simulink model "implementation_deploy_simulador"  (R2024b)
settings: configuration reference "Configuration" (kept outside this file)
undefined symbols (not defined in the file): aceleracao_lateral_max, constans_PID, desired_x, desired_y, DiscIntNeverNeededParam, max_velocity_longitudinal, pos_theta, pos_x, pos_y, vel_x
libraries: ros2lib x4, simulink_extras x1, drivingvehiclecontroller x1, slpidlib x1
settings Model: DataDictionary=mplementacao_deploy_simulador.sldd  Creator=helenamandl  LastModifiedBy=thailon
settings ConfigSetRef: SourceName=Configuration

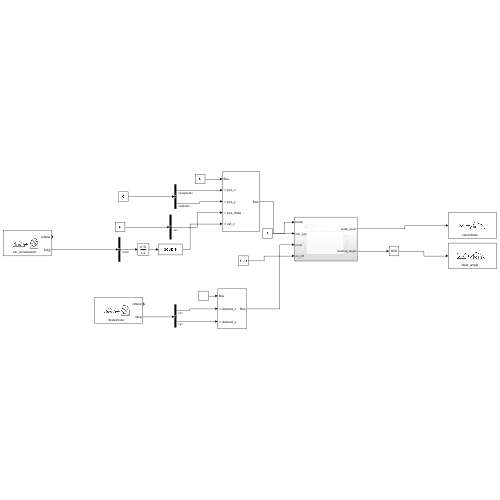
[thumbnail: Simulink's stored preview of the top-level diagram]
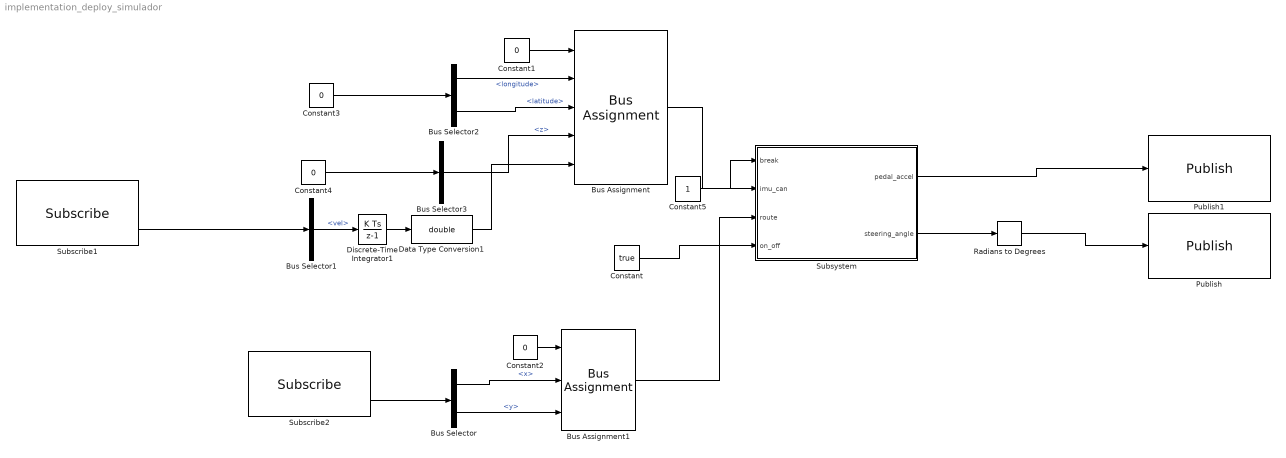
== system implementation_deploy_simulador ==
  Bus Assignment : BusAssignment  AssignedSignals=pos_x,pos_y,pos_theta,vel_x
  Bus Assignment1 : BusAssignment  AssignedSignals=desired_x,desired_y
  Bus Selector : BusSelector  OutputSignals=pose.position.x,pose.position.y
  Bus Selector1 : BusSelector  OutputSignals=vel
  Bus Selector2 : BusSelector  OutputSignals=longitude,latitude
  Bus Selector3 : BusSelector  OutputSignals=z
  Constant : Constant  Value=true  OutDataTypeStr=boolean
  Constant1 : Constant  Value=0  OutDataTypeStr=Bus: bus_imu
  Constant2 : Constant  Value=0  OutDataTypeStr=Bus: bus_route
  Constant3 : Constant  Value=0  OutDataTypeStr=Bus: bus_imu
  Constant4 : Constant  Value=0  OutDataTypeStr=Bus: bus_imu
  Constant5 : Constant
  Data Type Conversion1 : DataTypeConversion  OutDataTypeStr=double  SaturateOnIntegerOverflow=off  RndMeth=Floor
  Discrete-Time Integrator1 : DiscreteIntegrator  SampleTime=-1  ICPrevOutput=DiscIntNeverNeededParam  ICPrevScaledInput=DiscIntNeverNeededParam
  Publish : ros2lib/Publish  topicSource=Specify your own  topic=steer_angle  messageType=std_msgs/Float32  QOSHistory=Keep last  QOSDepth=1  QOSReliability=Reliable  QOSDurability=Volatile  QOSDeadline=Inf  QOSLifespan=Inf  QOSLiveliness=Automatic  QOSLeaseDuration=Inf  QOSAvoidROSNamespaceConventions=off
  Publish1 : ros2lib/Publish  topicSource=Specify your own  topic=velocidade  messageType=std_msgs/Float32  QOSHistory=Keep last  QOSDepth=1  QOSReliability=Reliable  QOSDurability=Volatile  QOSDeadline=Inf  QOSLifespan=Inf  QOSLiveliness=Automatic  QOSLeaseDuration=Inf  QOSAvoidROSNamespaceConventions=off
  Radians to Degrees : simulink_extras/Transformations/Radians to Degrees
  Subscribe1 : ros2lib/Subscribe  topicSource=Specify your own  topic=car_acceleration  messageType=std_msgs/Float32  sampleTime=ts_ros2  QOSHistory=Keep last  QOSDepth=10  QOSReliability=Reliable  QOSDurability=Volatile  QOSDeadline=Inf  QOSLifespan=Inf  QOSLiveliness=Automatic  QOSLeaseDuration=Inf  QOSAvoidROSNamespaceConventions=off
  Subscribe2 : ros2lib/Subscribe  topicSource=Specify your own  topic=/teste/route  messageType=geometry_msgs/PoseStamped  sampleTime=ts_ros2  QOSHistory=Keep last  QOSDepth=10  QOSReliability=Reliable  QOSDurability=Volatile  QOSDeadline=Inf  QOSLifespan=Inf  QOSLiveliness=Automatic  QOSLeaseDuration=Inf  QOSAvoidROSNamespaceConventions=off
  Subsystem : Subsystem
  wires:
  Subsystem/1(pedal_accel) -> Publish1/1
  Bus Assignment1/1 -> Subsystem/3(route)
  Constant/1 -> Subsystem/4(on_off)
  Bus Assignment/1 -> Subsystem/2(imu_can)
  Bus Selector/2 -> Bus Assignment1/3  "<y>"
  Bus Selector1/1 -> Discrete-Time Integrator1/1  "<vel>"
  Constant2/1 -> Bus Assignment1/1
  Constant5/1 -> Subsystem/1(break)
  Constant3/1 -> Bus Selector2/1
  Subscribe2/2 -> Bus Selector/1
  Subsystem/2(steering_angle) -> Radians to Degrees/1
  Constant4/1 -> Bus Selector3/1
  Data Type Conversion1/1 -> Bus Assignment/5
  Bus Selector/1 -> Bus Assignment1/2  "<x>"
  Constant1/1 -> Bus Assignment/1
  Bus Selector2/1 -> Bus Assignment/2  "<longitude>"
  Bus Selector2/2 -> Bus Assignment/3  "<latitude>"
  Bus Selector3/1 -> Bus Assignment/4  "<z>"
  Radians to Degrees/1 -> Publish/1
  Subscribe1/2 -> Bus Selector1/1
  Discrete-Time Integrator1/1 -> Data Type Conversion1/1

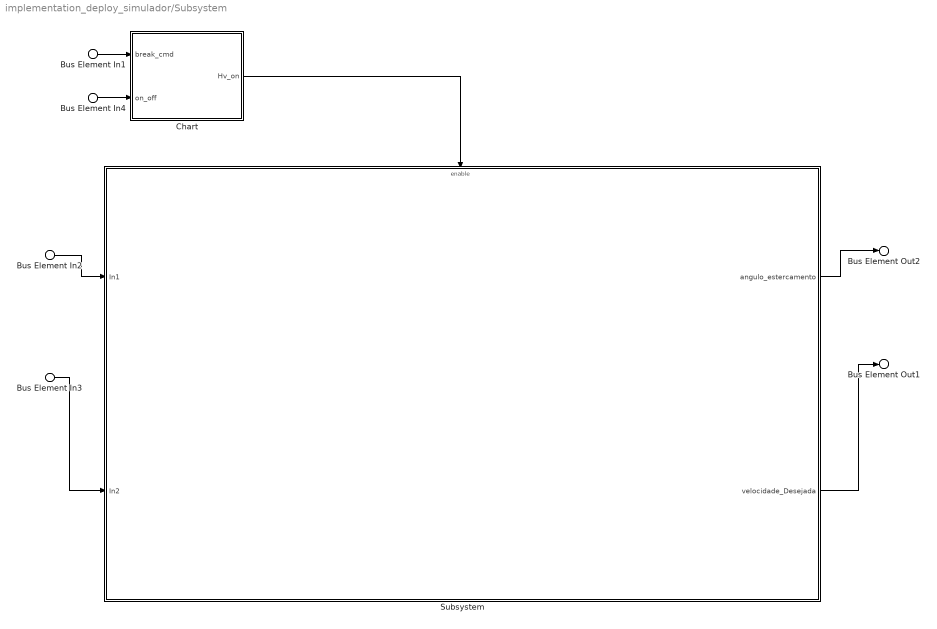
== system implementation_deploy_simulador/Subsystem ==
  Bus Element In1 : Inport  PortName=break
  Bus Element In2 : Inport  Port=2  PortName=imu_can
  Bus Element In3 : Inport  Port=3  PortName=route
  Bus Element In4 : Inport  Port=4  PortName=on_off
  Chart : Stateflow chart  TreatAsAtomicUnit=on
  Subsystem : Subsystem
  Bus Element Out1 : Outport  PortName=pedal_accel
  Bus Element Out2 : Outport  Port=2  PortName=steering_angle
  wires:
  Bus Element In1/1 -> Chart/1(break_cmd)
  Subsystem/1(angulo_estercamento) -> Bus Element Out2/1
  Subsystem/2(velocidade_Desejada) -> Bus Element Out1/1
  Chart/1(Hv_on) -> Subsystem/Enable
  Bus Element In4/1 -> Chart/2(on_off)
  Bus Element In2/1 -> Subsystem/1(In1)
  Bus Element In3/1 -> Subsystem/2(In2)

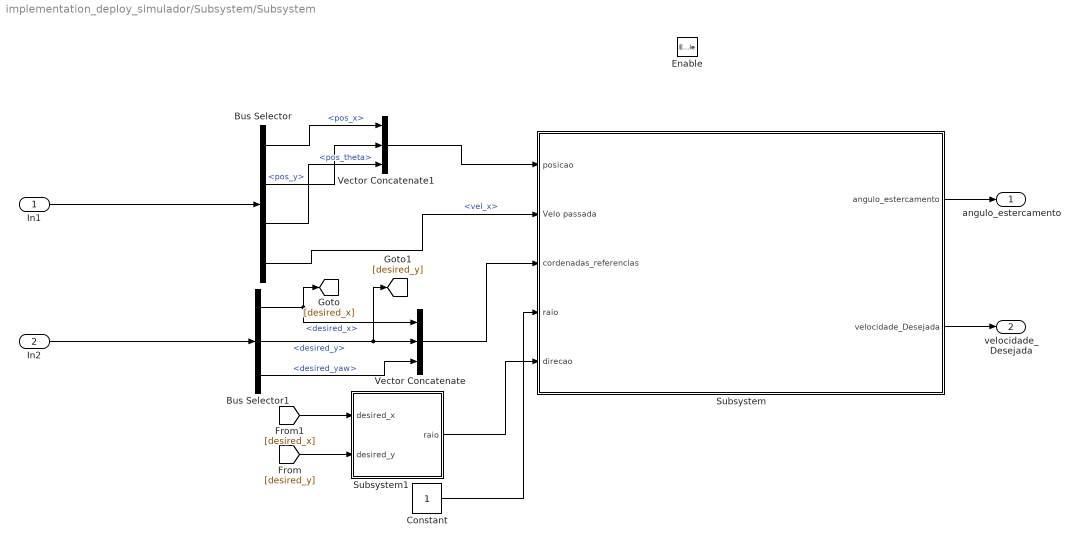
== system implementation_deploy_simulador/Subsystem/Subsystem ==
  In1 : Inport
  In2 : Inport  Port=2
  Enable : EnablePort
  Bus Selector : BusSelector  OutputSignals=pos_x,pos_y,pos_theta,vel_x
  Bus Selector1 : BusSelector  OutputSignals=desired_x,desired_y,desired_yaw
  Constant : Constant
  Subsystem : Subsystem
  Subsystem1 : Subsystem
  Vector Concatenate : Concatenate  NumInputs=3
  Vector Concatenate1 : Concatenate  NumInputs=3
  angulo_estercamento : Outport
  velocidade_Desejada : Outport  Port=2
  wires:
  Subsystem1/1(raio) -> Subsystem/5(direcao)
  [desired_y] -> Subsystem1/2(desired_y)
  Bus Selector/4 -> Subsystem/2(Velo passada)  "<vel_x>"
  Subsystem/1(angulo_estercamento) -> angulo_estercamento/1
  Bus Selector/1 -> Vector Concatenate1/1  "<pos_x>"
  Bus Selector1/1 -> Vector Concatenate/1, [desired_x]  "<desired_x>"
  Bus Selector/2 -> Vector Concatenate1/2  "<pos_y>"
  [desired_x] -> Subsystem1/1(desired_x)
  In1/1 -> Bus Selector/1
  Bus Selector1/2 -> Vector Concatenate/2, [desired_y]  "<desired_y>"
  Vector Concatenate/1 -> Subsystem/3(cordenadas_referencias)
  Bus Selector1/3 -> Vector Concatenate/3  "<desired_yaw>"
  In2/1 -> Bus Selector1/1
  Constant/1 -> Subsystem/4(raio)
  Bus Selector/3 -> Vector Concatenate1/3  "<pos_theta>"
  Subsystem/2(velocidade_Desejada) -> velocidade_Desejada/1
  Vector Concatenate1/1 -> Subsystem/1(posicao)

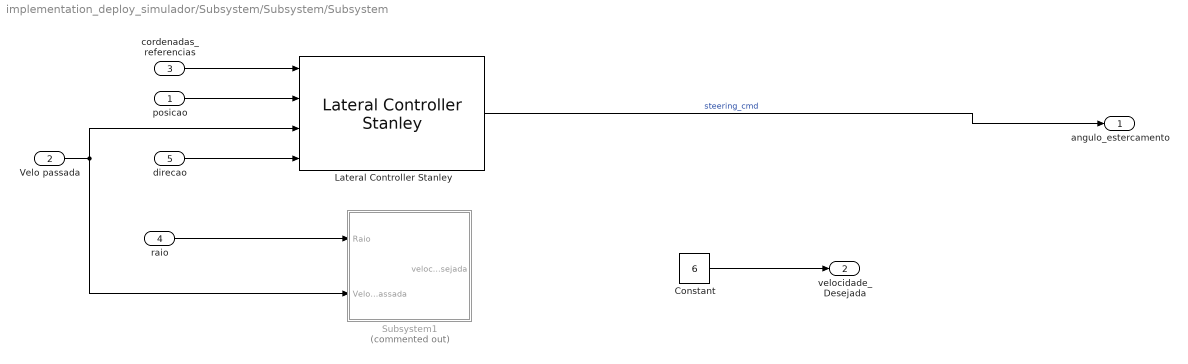
== system implementation_deploy_simulador/Subsystem/Subsystem/Subsystem ==
  posicao : Inport
  Velo passada : Inport  Port=2
  cordenadas_referencias : Inport  Port=3
  raio : Inport  Port=4
  direcao : Inport  Port=5
  Constant : Constant  Value=6
  Lateral Controller Stanley : drivingvehiclecontroller/Lateral Controller Stanley  ModelType=Kinematic bicycle model  PositionGainF=stanley_kpfw  PositionGainR=stanley_kprv  YawRateGain=1  DelayGain=0.2  VehicleMass=230  Lf=1.4  Lr=1.6  TireStiffness=12e3  Wheelbase=wheelbase  MaxSteeringAngle=max_steering_angle
  Subsystem1 : Subsystem  Commented=on
  angulo_estercamento : Outport  OutMax=[0]  PortDimensions=1
  velocidade_Desejada : Outport  Port=2
  wires:
  direcao/1 -> Lateral Controller Stanley/4
  posicao/1 -> Lateral Controller Stanley/2
  Lateral Controller Stanley/1 -> angulo_estercamento/1  "steering_cmd"
  cordenadas_referencias/1 -> Lateral Controller Stanley/1
  Velo passada/1 -> Subsystem1/2(Velo passada), Lateral Controller Stanley/3
  raio/1 -> Subsystem1/1(Raio)
  Constant/1 -> velocidade_Desejada/1

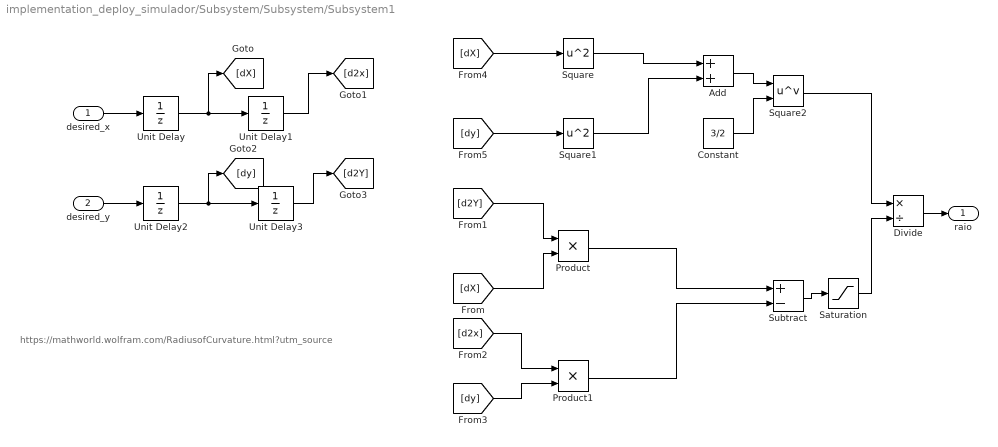
== system implementation_deploy_simulador/Subsystem/Subsystem/Subsystem1 ==
  note: https://mathworld.wolfram.com/RadiusofCurvature.html?utm_source
  desired_x : Inport
  desired_y : Inport  Port=2
  Add : Sum
  Constant : Constant  Value=3/2
  Divide : Product  Inputs=*/
  Product : Product
  Product1 : Product
  Saturation : Saturate  UpperLimit=10000  LowerLimit=0.00001
  Square : Math  Operator=square
  Square1 : Math  Operator=square
  Square2 : Math  Operator=pow
  Subtract : Sum  Inputs=+-
  Unit Delay{,1..3} (4 alike) : UnitDelay  SampleTime=-1  HasFrameUpgradeWarning=on
  raio : Outport
  wires:
  [dX] -> Square/1
  [d2x] -> Product1/1
  desired_x/1 -> Unit Delay/1
  [dy] -> Product1/2
  Product/1 -> Subtract/1
  Unit Delay1/1 -> [d2x]
  Add/1 -> Square2/1
  Unit Delay/1 -> [dX], Unit Delay1/1
  Square1/1 -> Add/2
  [d2Y] -> Product/1
  [dy] -> Square1/1
  Product1/1 -> Subtract/2
  [dX] -> Product/2
  desired_y/1 -> Unit Delay2/1
  Unit Delay2/1 -> [dy], Unit Delay3/1
  Constant/1 -> Square2/2
  Unit Delay3/1 -> [d2Y]
  Divide/1 -> raio/1
  Square2/1 -> Divide/1
  Subtract/1 -> Saturation/1
  Saturation/1 -> Divide/2
  Square/1 -> Add/1

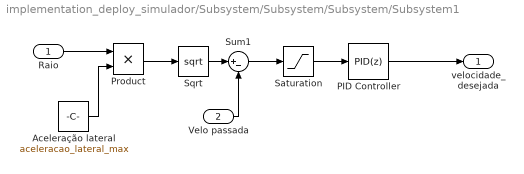
== system implementation_deploy_simulador/Subsystem/Subsystem/Subsystem/Subsystem1 ==
  Raio : Inport
  Velo passada : Inport  Port=2
  Aceleração lateral : Constant  Value=aceleracao_lateral_max
  PID Controller : slpidlib/PID Controller  Controller=PID  Form=Parallel  TimeDomain=Discrete-time  UseExternalTs=off  SampleTime=-1  IntegratorMethod=Forward Euler  FilterMethod=Forward Euler  ControllerParametersSource=internal  P=constans_PID(1)  I=constans_PID(2)  UseKiTs=off  D=constans_PID(3)  UseExternalDerivativeSource=off  N=constans_PID(4)  UseFilter=on  TunerSelectOption=Transfer Function Based (PID Tuner App)  InitialConditionSource=internal  InitialConditionForIntegrator=0  InitialConditionForFilter=0  DifferentiatorICPrevScaledInput=0  ExternalReset=none  TrackingMode=off  Kt=1  LimitOutput=off  SatLimitsSource=internal  UpperSaturationLimit=12  LowerSaturationLimit=-12  LinearizeAsGain=on  AntiWindupMode=none  Kb=1  LimitIntegrator=off  UpperIntegratorSaturationLimit=inf  LowerIntegratorSaturationLimit=-inf  POutMin=[]  POutMax=[]  IOutMin=[]  IOutMax=[]  DOutMin=[]  DOutMax=[]  NOutMin=[]  NOutMax=[]  SumOutMin=[]  SumOutMax=[]  SaturationOutMin=[]  SaturationOutMax=[]  PParamMin=[]  PParamMax=[]  IParamMin=[]  IParamMax=[]  DParamMin=[]  DParamMax=[]  NParamMin=[]  NParamMax=[]  KbParamMin=[]  KbParamMax=[]  KtParamMin=[]  KtParamMax=[]  KbOutMin=[]  KbOutMax=[]  KtOutMin=[]  KtOutMax=[]  IntegratorOutMin=[]  IntegratorOutMax=[]  FilterOutMin=[]  FilterOutMax=[]  SumI1OutMin=[]  SumI1OutMax=[]  SumI2OutMin=[]  SumI2OutMax=[]  SumI3OutMin=[]  SumI3OutMax=[]  SumI4OutMin=[]  SumI4OutMax=[]  SumDOutMin=[]  SumDOutMax=[]  DifferentiatorOutMin=[]  DifferentiatorOutMax=[]  FilterDiffOutCoefMin=[]  FilterDiffOutCoefMax=[]  ReciprocalOutMin=[]  ReciprocalOutMax=[]  SumDenOutMin=[]  SumDenOutMax=[]  SumNumOutMin=[]  SumNumOutMax=[]  DivideOutMin=[]  DivideOutMax=[]  UdiffTsProdOutMin=[]  UdiffTsProdOutMax=[]  NTsProdOutMin=[]  NTsProdOutMax=[]  UintegralTsProdOutMin=[]  UintegralTsProdOutMax=[]  UngainTsProdOutMin=[]  UngainTsProdOutMax=[]  ClampingZeroOutDataTypeStr=Inherit: Inherit via back propagation  ClampingZeroOutMin=[]  ClampingZeroOutMax=[]  FilterDenConstantOutDataTypeStr=Inherit: Inherit via back propagation  FilterDenConstantOutMin=[]  FilterDenConstantOutMax=[]  PCopyOutDataTypeStr=Inherit: Inherit via back propagation  PCopyOutMin=[]  PCopyOutMax=[]  NCopyOutDataTypeStr=Inherit: Inherit via back propagation  NCopyOutMin=[]  NCopyOutMax=[]  IntegratorContinuousStateAttributes=''  IntegratorStateMustResolveToSignalObject=off  IntegratorRTWStateStorageClass=Auto  FilterContinuousStateAttributes=''  FilterStateMustResolveToSignalObject=off  FilterRTWStateStorageClass=Auto  ParallelPVariant=InternalParameters  IdealPVariant=Disabled  IVariant=InternalParameters  DVariant=InternalParameters  IntegratorVariant=Discrete  SatVariant=Disabled  AWVariant=Passthrough  PCopyVariant=Disabled  TRVariant=Disabled  FdbkBlocksVariant=Forward  IdealPFdbkVariant=Disabled  SatFdbkVariant=Disabled  DerivativeFilterVariant=ForwardEulerFilter  NVariant=InternalParameters  NCopyVariant=Disabled  FilterICVariant=InternalICsFilter  IntegratorICVariant=InternalICs  ExternalResetVariant=Disabled  TRSumVariant=Passthrough  SumFdbkVariant=Disabled  SumVariant=Sum_PID  TsampFilterVariant=InternalTs  TsampNgainVariant=Passthrough  TsampIntegralVariant=Disabled_SignalSpec  ExternalSaturationOutDataTypeStr=Inherit: Same as second input  DerivativeSourceVariant=ErrorSignal  PreIntVariant=InternalPreInt
  Product : Product
  Saturation : Saturate  UpperLimit=max_velocity_longitudinal  LowerLimit=0
      settings: AttributesFormatString=Velocidade maxima do carro=%<UpperLimit>
  Sqrt : Sqrt
  Sum1 : Sum  Inputs=|+-
  velocidade_desejada : Outport
  wires:
  Saturation/1 -> PID Controller/1
  Sum1/1 -> Saturation/1
  PID Controller/1 -> velocidade_desejada/1
  Product/1 -> Sqrt/1
  Aceleração lateral/1 -> Product/2
  Sqrt/1 -> Sum1/1
  Raio/1 -> Product/1
  Velo passada/1 -> Sum1/2

== stateflow chart implementation_deploy_simulador/Subsystem/Chart ==
  state Idle
  state HV
    entry:
    Hv_on = 1;
  (default) -> Idle
  Idle -> HV : [on_off==true]
  HV -> Idle : [(on_off == false)]
  data: break_cmd input; on_off input; Hv_on output
